simulink model "RAKE_SS_4F_Rayleigh_2021b"  (R2021b)
settings: Solver=VariableStepDiscrete  StartTime=0.0  StopTime=inf  RelTol=1e-3  EnableMultiTasking=on
PreLoadFcn:
  | SNR=0;
  | a= [1/sqrt(2) 1/sqrt(20) 0 0];
values from neighbouring files (symbols this model uses):
  aest = input('Estimated four-path channel gains: ')    [run_RAKE_Rayleigh_2021b.m]    (also in run_RAKE_Rayleigh_2024b.m)
  c = input('Four-path channel gains: ')    [run_RAKE_Rayleigh_2021b.m]    (also in run_RAKE_Rayleigh_2024b.m)
  Nav = 4    [run_RAKE_Rayleigh_2021b.m]    (also in run_RAKE_Rayleigh_2024b.m)
  seed = input('Enter the last five digits of your student ID: ')    [run_OFDM_2011b.m]    (also in run_OFDM_2024b.m; run_RAKE_Rayleigh_2021b.m = input('Enter your student ID: '); run_RAKE_Rayleigh_2024b.m = input('Enter your student ID: '))
  Tf = 100    [run_RAKE_Rayleigh_2021b.m]    (also in run_RAKE_Rayleigh_2024b.m)
undefined symbols (not defined in the file or in its folder): DiscIntNeverNeededParam
libraries: simulink x4, commdigbbndpm3 x3, commseqgen3 x2, commrandsrc2 x1, commsink2 x1, commchan3 x1
settings Model: Creator=morelos_zaragoza  LastModifiedBy=14083
settings SolverCC: AlgebraicLoopSolver=TrustRegion
settings DataIOCC: LimitDataPoints=on  SaveFormat=Array  SignalLoggingSaveFormat=ModelDataLogs  ReturnWorkspaceOutputs=off
settings OptimizationCC: ExpressionDepthLimit=2147483647  InitFltsAndDblsToZero=on  LifeSpan=inf
settings DebuggingCC: SaveWithParameterizedLinksMsg=none  UnderspecifiedInitializationDetection=Classic  MergeDetectMultiDrivingBlocksExec=none  SignalResolutionControl=TryResolveAllWithWarning  SolverPrmCheckMsg=warning  MultiTaskDSMMsg=warning  MultiTaskCondExecSysMsg=none  FcnCallInpInsideContextMsg=warning  StateNameClashWarn=warning  SFUnexpectedBacktrackingDiag=warning  SFNoUnconditionalDefaultTransitionDiag=warning  SFExecutionAtInitializationDiag=none  SFMachineParentedDataDiag=warning  ArithmeticOperatorsInVariantConditions=warning
settings HardwareCC: ProdBitPerPointer=32  ProdBitPerSizeT=32  ProdBitPerPtrDiffT=32  ProdLargestAtomicFloat=None  ProdIntDivRoundTo=Undefined  ProdEndianess=Unspecified  ProdWordSize=32  ProdHWDeviceType=32-bit Generic
settings ModelReferenceCC: PropagateSignalLabelsOutOfModel=off
settings SFSimCC: SimUseLocalCustomCode=off  CustomCodeUndefinedFunction=UseInterfaceOnly
settings RTWCC: RTWUseLocalCustomCode=off
settings CodeAppCC: StateflowObjectComments=on
settings GRTTargetCC: TargetFcnLib=ansi_tfl_tmw.mat  TargetLangStandard=C89/C90 (ANSI)  CombineOutputUpdateFcns=off  GRTInterface=on
settings ConfigComp: CovMetricSettings=dw  CovSaveCumulativeToWorkspaceVar=on  CovSaveSingleToWorkspaceVar=on  CovExternalEMLEnable=off

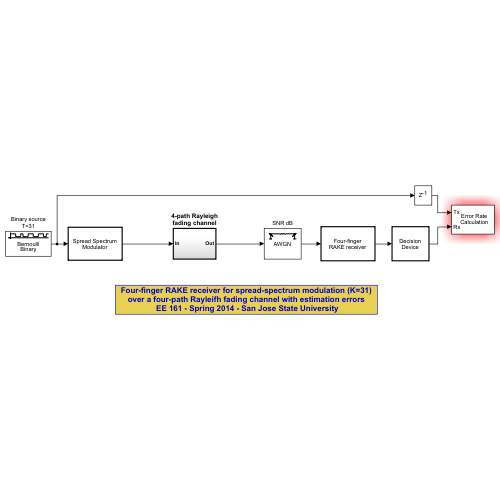
[thumbnail: Simulink's stored preview of the top-level diagram]
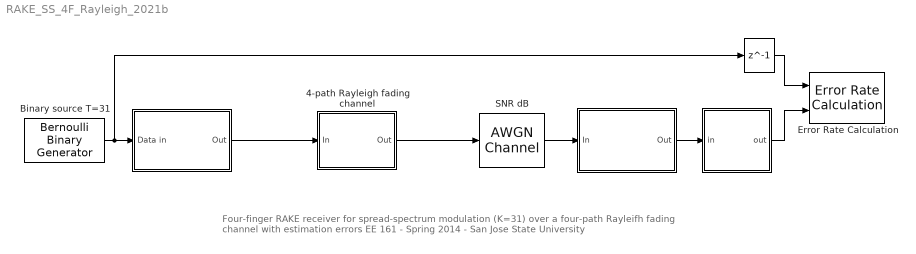
== system RAKE_SS_4F_Rayleigh_2021b ==
  note: Four-finger RAKE receiver for spread-spectrum modulation (K=31)
      | over a four-path Rayleifh fading channel with estimation errors
      | EE 161 - Spring 2014 - San Jose State University
  " " : Subsystem  TreatAsAtomicUnit=on
      mask Display: disp('Spread Spectrum\nModulator')
  "  " : Subsystem  TreatAsAtomicUnit=on
      mask Display: disp('Four-finger\nRAKE receiver')
  "   " : Delay  DelayLength=1  SampleTime=31
  "    " : Subsystem  TreatAsAtomicUnit=on
      mask Display: disp('Decision\nDevice')
  4-path Rayleigh fading channel : Subsystem  TreatAsAtomicUnit=on
  Binary source T=31 : commrandsrc2/Bernoulli Binary Generator  P=0.5  seed=61175  Ts=31  frameBased=off  sampPerFrame=1  orient=off  outDataType=double
      settings: SourceProductBaseCode=CM
  Error Rate Calculation : commsink2/Error Rate Calculation  N=0  st_delay=1  cp_mode=Entire frame  subframe=[]  PMode=Workspace  WsName=ErrorVec  RsMode2=off  stop=on  numErr=300  maxBits=Nsim
  SNR dB : commchan3/AWGN Channel  InputProcessing=Columns as channels (frame based)  seed=6713421  noiseMode="Signal to noise ratio  (SNR)"  EbNodB=SNR  EsNodB=SNR  SNRdB=SNR  bitsPerSym=1  Ps=1  Tsym=31  variance=1
  wires:
  " "/1(Out) -> 4-path Rayleigh fading channel/1(In)
  Binary source T=31/1 -> " "/1(Data in), "   "/1
  SNR dB/1 -> "  "/1(In)
  "  "/1(Out) -> "    "/1(in)
  "    "/1(out) -> Error Rate Calculation/2
  "   "/1 -> Error Rate Calculation/1
  4-path Rayleigh fading channel/1(Out) -> SNR dB/1

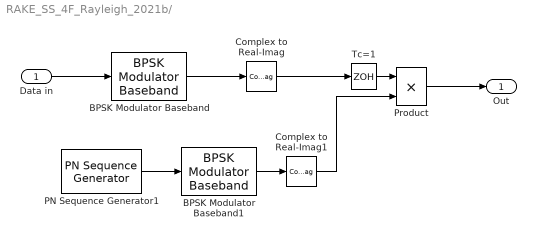
== system RAKE_SS_4F_Rayleigh_2021b/  ==
  Data in : Inport
  BPSK Modulator Baseband : commdigbbndpm3/BPSK Modulator Baseband  Ph=0  outDtype=double  outWordLen=16  outUDDataType=sfix(16)  outFracLenMode=Best precision  outFracLen=15  outDataTypeStr=double  outLastDataTypeStr=double
  BPSK Modulator Baseband1 : commdigbbndpm3/BPSK Modulator Baseband  Ph=0  outDtype=double  outWordLen=16  outUDDataType=sfix(16)  outFracLenMode=Best precision  outFracLen=15  outDataTypeStr=double  outLastDataTypeStr=double
  Complex to Real-Imag : ComplexToRealImag  Output=Real
  Complex to Real-Imag1 : ComplexToRealImag  Output=Real
  PN Sequence Generator1 : commseqgen3/PN Sequence Generator  poly="[1 0  0 1 0 1]"  ini_sta=[1 0 0 0 1]  outBitMaskSource=Dialog parameter  shift=0  outVarSiz=off  maxOutSizeMode=Dialog parameter  maxOutSize=[10 1]  Ts=1  sampPerFrame=1  reset=off  bitPackedOutputs=off  outDataType=double  numPackedBits=8  bitPackDataSigned=off  bitPackedOutDType=double
  Product : Product  SaturateOnIntegerOverflow=on  OutDataTypeStr=Inherit: Same as first input
  Tc=1 : ZeroOrderHold
  Out : Outport  VectorParamsAs1DForOutWhenUnconnected=off
  wires:
  PN Sequence Generator1/1 -> BPSK Modulator Baseband1/1
  BPSK Modulator Baseband1/1 -> Complex to Real-Imag1/1
  BPSK Modulator Baseband/1 -> Complex to Real-Imag/1
  Data in/1 -> BPSK Modulator Baseband/1
  Complex to Real-Imag1/1 -> Product/2
  Complex to Real-Imag/1 -> Tc=1/1
  Tc=1/1 -> Product/1
  Product/1 -> Out/1

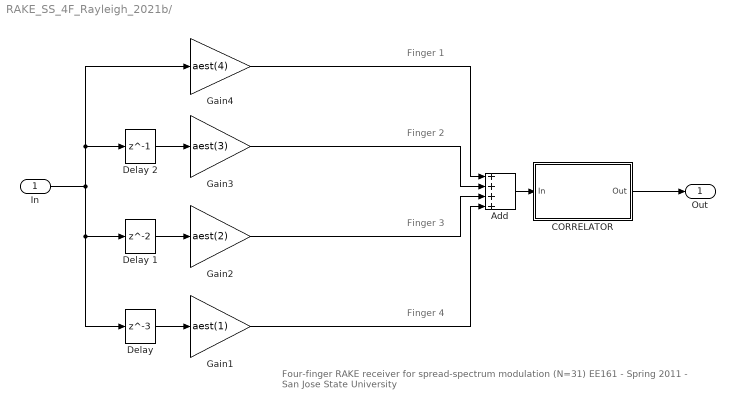
== system RAKE_SS_4F_Rayleigh_2021b/   ==
  note: Finger 1
  note: Finger 4
  note: Finger 2
  note: Finger 3
  note: Four-finger RAKE receiver for spread-spectrum modulation (N=31)
      | EE161 - Spring 2011 - San Jose State University
  In : Inport
  "   Delay " : Delay  DelayLength=3  SampleTime=1
  "   Delay 1" : Delay  SampleTime=1
  "   Delay 2" : Delay  DelayLength=1  SampleTime=1
  Add : Sum  Inputs=++++
  CORRELATOR : Subsystem  TreatAsAtomicUnit=on
  "Gain1 " : Gain  Gain=aest(1)
  "Gain2 " : Gain  Gain=aest(2)
  "Gain3 " : Gain  Gain=aest(3)
  "Gain4 " : Gain  Gain=aest(4)
  Out : Outport  VectorParamsAs1DForOutWhenUnconnected=off
  wires:
  "Gain4 "/1 -> Add/1
  "   Delay "/1 -> "Gain1 "/1
  Add/1 -> CORRELATOR/1(In)
  CORRELATOR/1(Out) -> Out/1
  "   Delay 1"/1 -> "Gain2 "/1
  "   Delay 2"/1 -> "Gain3 "/1
  In/1 -> "Gain4 "/1, "   Delay 2"/1, "   Delay 1"/1, "   Delay "/1
  "Gain3 "/1 -> Add/2
  "Gain2 "/1 -> Add/3
  "Gain1 "/1 -> Add/4

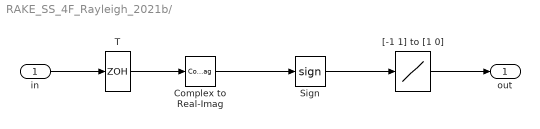
== system RAKE_SS_4F_Rayleigh_2021b/     ==
  in : Inport
  Complex to Real-Imag : ComplexToRealImag  Output=Real
  Sign : Signum
  T : ZeroOrderHold  SampleTime=31
  "[-1 1] to [1 0]" : Lookup  InputValues=[-1 1]  Table=[1 0]  OutDataTypeStr=double  SaturateOnIntegerOverflow=on
  out : Outport  VectorParamsAs1DForOutWhenUnconnected=off
  wires:
  Sign/1 -> "[-1 1] to [1 0]"/1
  Complex to Real-Imag/1 -> Sign/1
  T/1 -> Complex to Real-Imag/1
  in/1 -> T/1
  "[-1 1] to [1 0]"/1 -> out/1

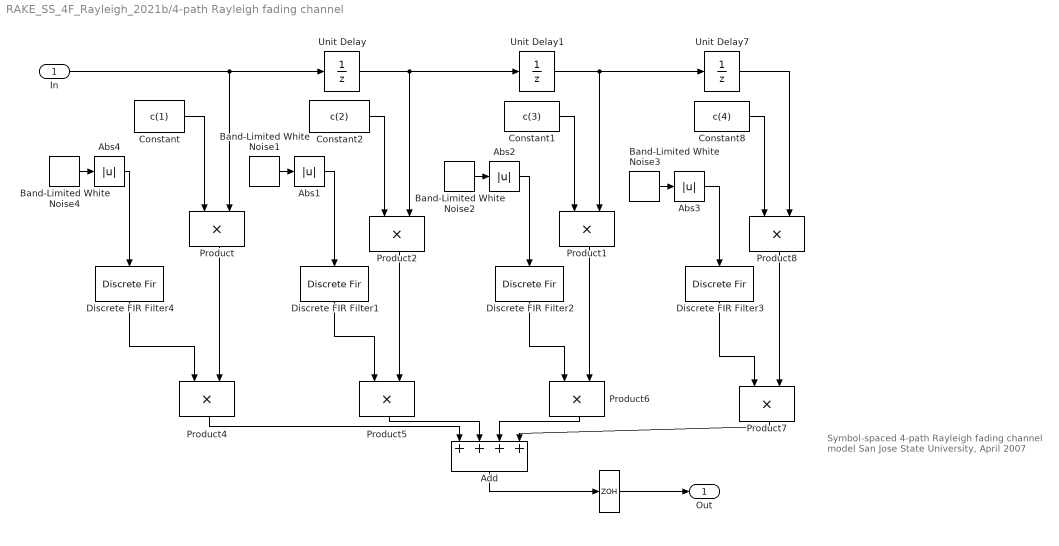
== system RAKE_SS_4F_Rayleigh_2021b/4-path Rayleigh fading channel ==
  note: Symbol-spaced 4-path
      | Rayleigh fading channel model
      | San Jose State University, April 2007
  In : Inport
  "       " : ZeroOrderHold
  Abs{1..4} (4 alike) : Abs
  Add : Sum  Inputs=++++
  Band-Limited White Noise1 : simulink/Sources/Band-Limited White Noise  Cov=[1]  Ts=Tf  seed=[seed+100]
  Band-Limited White Noise2 : simulink/Sources/Band-Limited White Noise  Cov=[1]  Ts=Tf  seed=[seed+243]
  Band-Limited White Noise3 : simulink/Sources/Band-Limited White Noise  Cov=[1]  Ts=Tf  seed=[seed+643]
  Band-Limited White Noise4 : simulink/Sources/Band-Limited White Noise  Cov=[1]  Ts=Tf  seed=[seed+1]
  Constant : Constant  Value=c(1)
  Constant1 : Constant  Value=c(3)
  Constant2 : Constant  Value=c(2)
  Constant8 : Constant  Value=c(4)
  Discrete FIR Filter{1..4} (4 alike) : DiscreteFir  Coefficients=[ones(1,Nav)]/sqrt(Nav)
  Product{,1..2,4..8} (8 alike) : Product  SaturateOnIntegerOverflow=on  OutDataTypeStr=Inherit: Same as first input
  Unit Delay : UnitDelay  HasFrameUpgradeWarning=on
  Unit Delay1 : UnitDelay  HasFrameUpgradeWarning=on
  Unit Delay7 : UnitDelay  HasFrameUpgradeWarning=on
  Out : Outport  VectorParamsAs1DForOutWhenUnconnected=off
  wires:
  In/1 -> Unit Delay/1, Product/2
  Unit Delay/1 -> Unit Delay1/1, Product2/2
  Unit Delay7/1 -> Product8/2
  Constant/1 -> Product/1
  Constant8/1 -> Product8/1
  "       "/1 -> Out/1
  Unit Delay1/1 -> Product1/2, Unit Delay7/1
  Constant1/1 -> Product1/1
  Constant2/1 -> Product2/1
  Add/1 -> "       "/1
  Product/1 -> Product4/2
  Product2/1 -> Product5/2
  Product1/1 -> Product6/2
  Product8/1 -> Product7/2
  Product4/1 -> Add/1
  Product5/1 -> Add/2
  Product6/1 -> Add/3
  Product7/1 -> Add/4
  Discrete FIR Filter1/1 -> Product5/1
  Discrete FIR Filter2/1 -> Product6/1
  Discrete FIR Filter3/1 -> Product7/1
  Band-Limited White Noise1/1 -> Abs1/1
  Abs1/1 -> Discrete FIR Filter1/1
  Band-Limited White Noise2/1 -> Abs2/1
  Abs2/1 -> Discrete FIR Filter2/1
  Band-Limited White Noise3/1 -> Abs3/1
  Abs3/1 -> Discrete FIR Filter3/1
  Abs4/1 -> Discrete FIR Filter4/1
  Band-Limited White Noise4/1 -> Abs4/1
  Discrete FIR Filter4/1 -> Product4/1

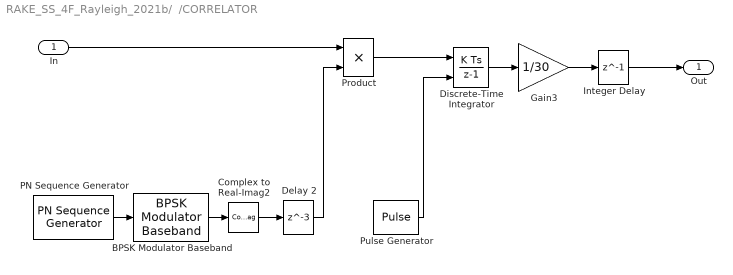
== system RAKE_SS_4F_Rayleigh_2021b/  /CORRELATOR ==
  In : Inport
  BPSK Modulator Baseband : commdigbbndpm3/BPSK Modulator Baseband  Ph=0  outDtype=double  outWordLen=16  outUDDataType=sfix(16)  outFracLenMode=Best precision  outFracLen=15  outDataTypeStr=double  outLastDataTypeStr=double
  Complex to Real-Imag2 : ComplexToRealImag  Output=Real
  Delay 2 : Delay  DelayLength=3  SampleTime=1
  Discrete-Time Integrator : DiscreteIntegrator  ExternalReset=level  UpperSaturationLimit=1  LowerSaturationLimit=0  ICPrevOutput=DiscIntNeverNeededParam  ICPrevScaledInput=DiscIntNeverNeededParam
  Gain3 : Gain  Gain=1/30
  Integer Delay : Delay  DelayLength=1  SampleTime=1
  PN Sequence Generator : commseqgen3/PN Sequence Generator  poly="[1 0  0 1 0 1]"  ini_sta=[1 0 0 0 1]  outBitMaskSource=Dialog parameter  shift=0  outVarSiz=off  maxOutSizeMode=Dialog parameter  maxOutSize=[10 1]  Ts=1  sampPerFrame=1  reset=off  bitPackedOutputs=off  outDataType=double  numPackedBits=8  bitPackDataSigned=off  bitPackedOutDType=double
  Product : Product  SaturateOnIntegerOverflow=on  OutDataTypeStr=Inherit: Same as first input
  Pulse Generator : DiscretePulseGenerator  Period=31
  Out : Outport  VectorParamsAs1DForOutWhenUnconnected=off
  wires:
  Pulse Generator/1 -> Discrete-Time Integrator/2
  PN Sequence Generator/1 -> BPSK Modulator Baseband/1
  BPSK Modulator Baseband/1 -> Complex to Real-Imag2/1
  Complex to Real-Imag2/1 -> Delay 2/1
  Product/1 -> Discrete-Time Integrator/1
  Delay 2/1 -> Product/2
  In/1 -> Product/1
  Discrete-Time Integrator/1 -> Gain3/1
  Gain3/1 -> Integer Delay/1
  Integer Delay/1 -> Out/1
